simulink library "isl_connect"  (R2024b)
settings: Solver=ode45  StartTime=0.0  StopTime=10.0  RelTol=1e-3  EnableMultiTasking=on
undefined symbols (not defined in the file or in its folder): g_ISLNotConnect, g_ISLStore, g_ISLXMLFile, islconnector, parameters
Description:
  | ISL Connectors
settings Model: Creator=thier  LastModifiedBy=thier
settings SolverCC: AlgebraicLoopSolver=TrustRegion
settings DataIOCC: LimitDataPoints=on  SaveFormat=Array  ReturnWorkspaceOutputs=off
settings OptimizationCC: LifeSpan=inf
settings DebuggingCC: UnconnectedInputMsg=warning  UnconnectedOutputMsg=warning  UnconnectedLineMsg=warning  SFUnexpectedBacktrackingDiag=warning  SFNoUnconditionalDefaultTransitionDiag=warning  SFExecutionAtInitializationDiag=none  ArithmeticOperatorsInVariantConditions=warning
settings HardwareCC: ProdBitPerPointer=32  ProdBitPerSizeT=32  ProdBitPerPtrDiffT=32  ProdLargestAtomicFloat=None  ProdIntDivRoundTo=Undefined  ProdEndianess=Unspecified  ProdWordSize=32  ProdHWDeviceType=32-bit Generic
settings ModelReferenceCC: PropagateSignalLabelsOutOfModel=off
settings SFSimCC: SimUseLocalCustomCode=off  CustomCodeUndefinedFunction=UseInterfaceOnly
settings RTWCC: RTWUseLocalCustomCode=off  GPUComputeCapability=3.5
settings CodeAppCC: StateflowObjectComments=on
settings GRTTargetCC: TargetLangStandard=C89/C90 (ANSI)
settings ConfigComp: CovMetricSettings=dw  CovSaveCumulativeToWorkspaceVar=on  CovSaveSingleToWorkspaceVar=on  CovExternalEMLEnable=off

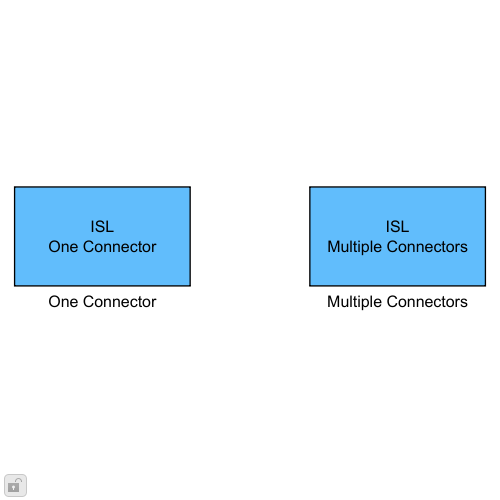
[thumbnail: Simulink's stored preview of the top-level diagram]
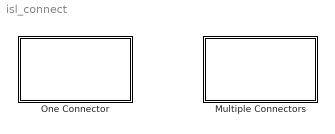
== system isl_connect ==
  Multiple Connectors : Subsystem
      mask Display: disp('ISL\nMultiple Connectors')
  One Connector : Subsystem
      mask Display: disp('ISL\nOne Connector')

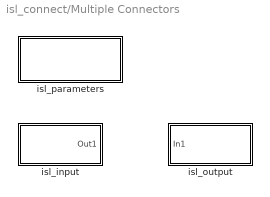
== system isl_connect/Multiple Connectors ==
  isl_input : Subsystem  mask(ISL Input){bSetStepSize=off, dStepSize=0.0, isltype=islin}
      mask prompts: bSetStepSize "Set step size"; dStepSize "Step size:"
      mask help:
      | The ISL input component is used to read data from the bus.
      | Multiple instances of the block are allowed.
      mask Help:
      | The ISL input component is used to read data from the bus.
      | Multiple instances of the block are allowed.
      mask Callback bSetStepSize:
      | en = get_param(gcb,'MaskVisibilities');
      | switch get_param(gcb,'bSetStepSize')
      |     case 'on'
      |         en{2} = 'on';
      |     case 'off'
      |         en{2} = 'off';
      |     otherwise
      |         en{2} = 'off';
      | end
      | set_param(gcb,'MaskVisibilities',en);
      mask Display: disp('ISL\nInput')
  isl_output : Subsystem  mask(ISL Output){bSetStepSize=off, dStepSize=0.0, dInitialStep=1e-6, isltype=islout}
      mask prompts: bSetStepSize "Set step size"; dStepSize "Step size:"; dInitialStep "Initial step:"
      mask help:
      | The ISL output component is used to write data to the bus.
      | Multiple instances of the block are allowed.
      mask Help:
      | The ISL output component is used to write data to the bus.
      | Multiple instances of the block are allowed.
      mask Callback bSetStepSize:
      | en = get_param(gcb,'MaskVisibilities');
      | switch get_param(gcb,'bSetStepSize')
      |     case 'on'
      |         en{2} = 'on';
      |         en{3} = 'on';
      |     case 'off'
      |         en{2} = 'off';
      |         en{3} = 'on';
      |     otherwise
      |         en{2} = 'off';
      |         en{3} = 'on';
      | end
      | set_param(gcb,'MaskVisibilities',en);
      mask Display: disp('ISL\nOutput')
  isl_parameters : Subsystem  InitFcn=|  mask{sXMLFile=, islconnecttype=parameters, bStore=off, bNotConnect=off}
      | g_ISLXMLFile = get_param(gcb, 'sXMLFile');
      | g_ISLStore = double(strcmp(get_param(gcb, 'bStore'), 'on'));
      | g_ISLNotConnect = double(strcmp(get_param(gcb, 'bNotConnect'), 'on'));
      mask prompts: sXMLFile "XML file"; islconnecttype "Type"; bStore "Store data"; bNotConnect "Do not connect ISL"
      mask DialogControl sXMLFile Tooltip: Relative path to an XML file
      mask DialogControl OptionsContainer Prompt: Options
      mask DialogControl bStore Tooltip: Check the box to store ISL data
      mask DialogControl bNotConnect Tooltip: Check the box to run out of the co-simulation
      mask Display: disp('ISL\nParameters')

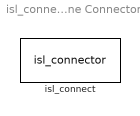
== system isl_connect/One Connector ==
  isl_connect : S-Function  FunctionName=isl_connector  Parameters=sXMLFile,bStore,bNotConnect,dInitialStep  SFunctionDeploymentMode=off  EnableBusSupport=off  mask(ISL connector v1.0){sXMLFile=, dInitialStep=1e-6, islconnecttype=islconnector, bStore=off, bNotConnect=off}
      mask prompts: sXMLFile "XML File:"; dInitialStep "Initial step:"; islconnecttype "Type"; bStore "Store data"; bNotConnect "Do not connect to ISL"
      mask help:
      | ISL connector connects Simulink variables to the ISL co-simulation bus. To setup the connector, specify a valid FMX file, and session name.
      |
      | IMPORTANT NOTE: Only one instance is allowed.
      mask Help:
      | ISL connector connects Simulink variables to the ISL co-simulation bus.
      | To setup the connector, specify a valid FMX file.
      | 
      | IMPORTANT NOTE: Only one instance is allowed.
      mask DialogControl OptionsContainer Prompt: Options
      mask Display: disp('ISL\nConnector 1.0')

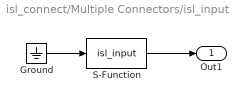
== system isl_connect/Multiple Connectors/isl_input ==
  Ground : Ground
  S-Function : S-Function  FunctionName=isl_input  Parameters=g_ISLXMLFile,g_ISLStore,g_ISLNotConnect,bSetStepSize,dStepSize  SFunctionDeploymentMode=off  EnableBusSupport=off
  Out1 : Outport
  wires:
  Ground/1 -> S-Function/1
  S-Function/1 -> Out1/1

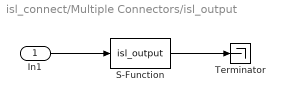
== system isl_connect/Multiple Connectors/isl_output ==
  In1 : Inport
  S-Function : S-Function  FunctionName=isl_output  Parameters=g_ISLXMLFile,g_ISLStore,g_ISLNotConnect,bSetStepSize,dStepSize,dInitialStep  SFunctionDeploymentMode=off  EnableBusSupport=off
  Terminator : Terminator
  wires:
  S-Function/1 -> Terminator/1
  In1/1 -> S-Function/1

== system isl_connect/Multiple Connectors/isl_parameters ==
